simulink model "testBufferStorage3pt"  (R2018b)
settings: Solver=ode23  StartTime=0.0  StopTime=7000  MaxStep=300  RelTol=1e-3  EnableMultiTasking=on
undefined symbols (not defined in the file or in its folder): path_carnot
libraries: carnot x21, SignalEditorBlockLib x1
settings Model: Creator=drhf  LastModifiedBy=drhf
settings DataIOCC: LimitDataPoints=on  SaveFormat=Array
settings OptimizationCC: ExpressionDepthLimit=2147483647  LifeSpan=inf
settings DebuggingCC: UnderspecifiedInitializationDetection=Classic  MergeDetectMultiDrivingBlocksExec=none  SolverPrmCheckMsg=warning  StateNameClashWarn=warning  SFUnexpectedBacktrackingDiag=warning  SFNoUnconditionalDefaultTransitionDiag=warning  SFExecutionAtInitializationDiag=none
settings HardwareCC: ProdBitPerPointer=32  ProdBitPerSizeT=32  ProdBitPerPtrDiffT=32  ProdLargestAtomicFloat=None  ProdIntDivRoundTo=Undefined  ProdEndianess=Unspecified  ProdWordSize=32  ProdHWDeviceType=32-bit Generic
settings ModelReferenceCC: PropagateSignalLabelsOutOfModel=off
settings SFSimCC: SimUseLocalCustomCode=off
settings RTWCC: RTWUseLocalCustomCode=off
settings CodeAppCC: StateflowObjectComments=on
settings GRTTargetCC: TargetLangStandard=C89/C90 (ANSI)  GeneratePreprocessorConditionals=Disable all  CombineOutputUpdateFcns=off  GRTInterface=on
settings ConfigComp: CovMetricSettings=dw  CovHtmlReporting=on  CovSaveCumulativeToWorkspaceVar=on  CovSaveSingleToWorkspaceVar=on  CovExternalEMLEnable=off

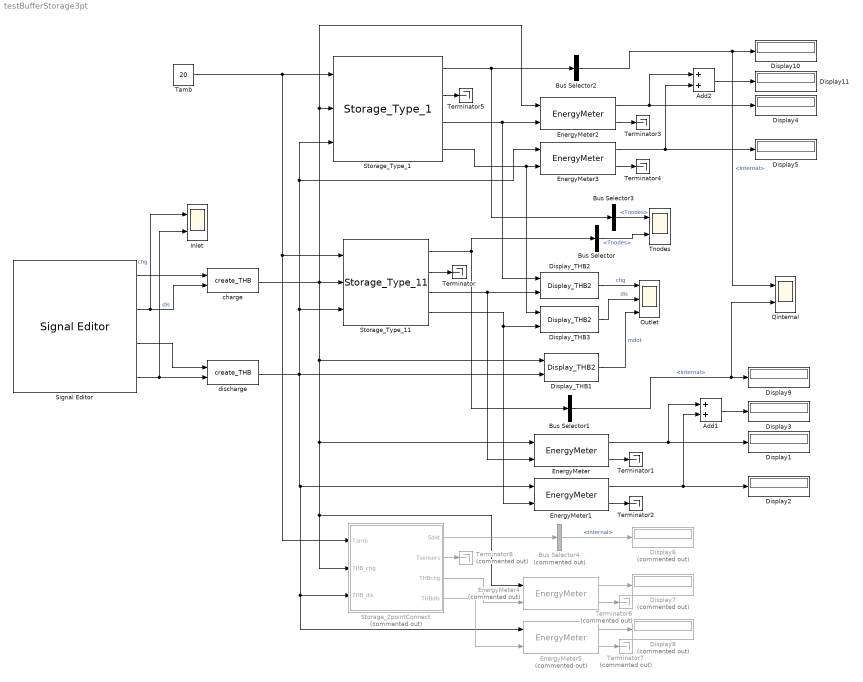
== system testBufferStorage3pt ==
  Add1 : Sum  Inputs=2
  Add2 : Sum  Inputs=2
  Bus Selector : BusSelector  OutputSignals=Tnodes
  Bus Selector1 : BusSelector  OutputSignals=energy.internal
  Bus Selector2 : BusSelector  OutputSignals=energy.internal
  Bus Selector3 : BusSelector  OutputSignals=Tnodes
  Bus Selector4 : BusSelector  Commented=on  OutputSignals=energy.internal
  Display{1..5,9..11} (8 alike) : Display
  Display6 : Display  Commented=on
  Display7 : Display  Commented=on
  Display8 : Display  Commented=on
  Display_THB1 : carnot/Outputs/Display_THB2  t=off  m=on  p=off  id=off  mix=off  d=off
      settings: SourceProductName=Carnot
  Display_THB2 : carnot/Outputs/Display_THB2  t=on  m=off  p=off  id=off  mix=off  d=off
      settings: SourceProductName=Carnot
  Display_THB3 : carnot/Outputs/Display_THB2  t=on  m=off  p=off  id=off  mix=off  d=off
      settings: SourceProductName=Carnot
  EnergyMeter{,1..3} (4 alike) : carnot/Control/EnergyMeter
      settings: SourceProductName=Carnot
  EnergyMeter4 : carnot/Control/EnergyMeter  Commented=on
      settings: SourceProductName=Carnot
  EnergyMeter5 : carnot/Control/EnergyMeter  Commented=on
      settings: SourceProductName=Carnot
  Inlet : Scope  NumInputPorts=2
  Outlet : Scope  NumInputPorts=3
  Qinternal : Scope  NumInputPorts=2
  Signal Editor : SignalEditorBlockLib/Signal Editor  FileName=storage3point_TestScenario.mat  ActiveScenario=Scenario  ActiveSignal=TDis  IsBus=off  OutputBusObjectStr=Bus: BusObject  SampleTime=0  ZeroCross=off  OutputAfterFinalValue=Setting to zero  Unit=inherit
  Storage_2pointConnect : Subsystem  Commented=on  mask(Buffer storage tank){t0=10, hgt=1.7684, stgtype=1, tini=[10 10 10 10 10 10 10 10 10 10], mpts=[1 2 3 4 5 6 7 8 9 10], PathName=fullfile(path_carnot('libsl'),'Storage','Thermal','Storage_Type_1','parameter_set'), FileName='StorageType1_500_L.mat', userPath=off, userParam=off, uwall=1, ubot=1, utop=1, axcond=1, volume=0.5, dia=0.6, standing=standing cylinder, nodes=10, mpoints=10, Tsensor=0.5, pipe1inlet=1, pipe1outlet=0, pipe1dia=0.03, pipe2inlet=0, pipe2outlet=1, pipe2dia=0.03}
      mask prompts: t0 "Initial temperature (vector or scalar) in °C"; hgt "Height of storage in m"; stgtype "Storage Type (0..5)"; tini "Start temperatures of nodes in °C"; mpts "Index to measured nodes"; PathName "Path"; FileName "Parameter set"; userPath "Edit path and name of parameter set"; userParam "User defined parameters"; uwall "Heat transfer coefficient to ambient [W/m²K]"; ubot "Heat transfer coefficient to ambient bottom [W/m²K]"; utop "Heat transfer coefficient to ambient top [W/m²K]"; axcond "Effective thermal conductivity [W/m/K]"; volume "Volume [m³]"; dia "Diameter [m]"; standing "Position"; nodes "Number of nodes"; mpoints "Number of node temperatures (for display)"; Tsensor "Temperature sensor position (0..1, 0 = bottom, 1 = top)"; pipe1inlet "relative height of inlet, range from 0 (= bottom) to 1 (= top)"; pipe1outlet "relative height of outlet, range from 0 (= bottom) to 1 (= top)"; pipe1dia "Diameter of pipe in m"; pipe2inlet "relative height of inlet, range from 0 (= bottom) to 1 (= top)"; pipe2outlet "relative height of outlet, range from 0 (= bottom) to 1 (= top)"; pipe2dia "Diameter of pipe in m"
      mask help:
      | Buffer storage for heating circuits. The storage model has the following components (with their typical position):
      | - one pipe connection for discharging (total height)
      | - one pipe connection for charging (total height)
      mask init:
      | [ok, param] = CarnotCallbacks_StorageConf('SetParam',stgtype,gcbh,PathName,FileName);
      mask Help: web(fullfile(path_carnot('help'),'Storage_Type_N.html'),'-helpbrowser')
      mask TypeOptions hgt: Pipe_Connection_1/hgt | Pipe_Connection_2/hgt
      mask TypeOptions stgtype: CreateSdat/stgtype
      mask TypeOptions tini: sfun_storageTnodes/tini
      mask TypeOptions mpts: select_T/Indices
      mask Callback userPath: [ok, param] = CarnotCallbacks_StorageConf('UserEdit',1,gcbh);
      mask Callback userParam: [ok, param] = CarnotCallbacks_StorageConf('UserEdit',1,gcbh);
      mask TypeOptions uwall: sfun_storageTnodes/uloss
      mask TypeOptions ubot: sfun_storageTnodes/ubot
      mask TypeOptions utop: sfun_storageTnodes/utop
      mask TypeOptions axcond: sfun_storageTnodes/cond
      mask TypeOptions volume: sfun_storageTnodes/volume | CreateSdat/volume
      mask TypeOptions dia: sfun_storageTnodes/dia | Pipe_Connection_1/dstg | Pipe_Connection_2/dstg
      mask TypeOptions standing: sfun_storageTnodes/standing
      mask TypeOptions nodes: sfun_storageTnodes/nodes | select_T/InputPortWidth | HX_EN12977_1/nodes | HX_EN12977_2/nodes | HX_EN12977_3/nodes | Pipe_Connection_1/nodes | Pipe_Connection_2/nodes | Pipe_Connection_3/nodes
      mask TypeOptions Tsensor: T_Sensor_Surface/pos
      mask TypeOptions pipe1inlet: Pipe_Connection_1/h_in
      mask TypeOptions pipe1outlet: Pipe_Connection_1/h_out
      mask TypeOptions pipe1dia: Pipe_Connection_1/dpipe
      mask TypeOptions pipe2inlet: Pipe_Connection_2/h_in
      mask TypeOptions pipe2outlet: Pipe_Connection_2/h_out
      mask TypeOptions pipe2dia: Pipe_Connection_2/dpipe
      mask DialogControl Container14 Prompt: Infos
      mask DialogControl ParameterGroupVar Prompt: Picking a parameter set
      mask DialogControl Control3 Prompt: Carnot public data
      mask DialogControl Control3 Callback: [ok, file] = CarnotCallbacks_StorageConf('GetFilename',1,gcbh,'public');
      mask DialogControl Control4 Prompt: Carnot internal data
      mask DialogControl Control4 Callback: [ok, file] = CarnotCallbacks_StorageConf('GetFilename',1,gcbh,'internal');
      mask DialogControl Control2 Prompt: Selected path
      mask DialogControl Control2 Callback: [ok, file] = CarnotCallbacks_StorageConf('GetFilename',1,gcbh,'selected');
      mask DialogControl Container4 Prompt: Parameter values
      mask DialogControl Container6 Prompt: Storage
      mask DialogControl Container8 Prompt: Connections
      mask DialogControl Container9 Prompt: Charging pipe
      mask DialogControl Container12 Prompt: Discharging pipe
      mask DialogControl Control6 Prompt: Save in Carnot internal data
      mask DialogControl Control6 Callback: [ok, param] = CarnotCallbacks_StorageConf('SaveFilename',1,gcbh,'internal','STG');
      mask DialogControl Control5 Prompt: Save in selected path
      mask DialogControl Control5 Callback: [ok, param] = CarnotCallbacks_StorageConf('SaveFilename',1,gcbh,'selected','STG');
      mask Display:
      | % user defined picture file
      | namestr = ['Storage_Type_', num2str(get_param(gcb,'stgtype'))];
      | picfile = fullfile(path_carnot('intlibsl'), 'Storage','Thermal', ...
      |     namestr,'parameter_set', [namestr, '.jpg']);
      | 
      | % show internal picture if defined
      | pic = false;
      | if  ~BlockIsInCarnotLibrary       % if not located in library
      |     if exist(picfile, 'file')
      |         image(imread(picfile), [0.25, 0, 0.45, 1])
      |         set_param(gcb, 'BackgroundColor', 'White')
      |         pic = true;
      |     end
      | end
      | 
      | % show public picture
      | if ~pic
      |     set_param(gcb, 'BackgroundColor', 'Red')
      | %     plot([40,30,30,40,60,70,70,60,40]/120+0.1,[90,80,10,0,0,10,80,90,90]/110+0.05, ...
      | %         [80,20]/120+0.1,[100,100]/110+0.05, ...
      | %         [50,50]/120+0.1,[90,100]/110+0.05, ...
      | %         [30,20]/120+0.1,[13,13]/110+0.05, ...
      | %         [80,70]/120+0.1,[13,13]/110+0.05)
      |       plot([40,30,30,40,60,70,70,60,40]/120+0.1,[90,80,20,10,10,20,80,90,90]/110+0.05, ...
      |            [80,20]/120+0.1,[100,100]/110+0.05, ...
      |            [50,50]/120+0.1,[90,100]/110+0.05, ...
      |            [80,20]/120+0.1,[0,0]/110+0.05, ...
      |            [50,50]/120+0.1,[0,10]/110+0.05)
      | end
  Storage_Type_1 : carnot/Storage/Thermal/Storage_Type_1  t0=10  hgt=1.7684  stgtype=1  tini=[10 10 10 10 10 10 10 10 10 10]  mpts=[1 2 3 4 5 6 7 8 9 10]  PathName=fullfile(path_carnot('libsl'),'Storage','Thermal','Storage_Type_1','parameter_set')  FileName='<user defined>'  userPath=off  userParam=on  uwall=1  ubot=1  utop=1  axcond=1  volume=0.5  dia=0.6  standing=standing cylinder  nodes=10  mpoints=10  Tsensor=0.5  pipe1inlet=1  pipe1outlet=0  pipe1dia=0.03  pipe2inlet=0.1  pipe2outlet=1  pipe2dia=0.03
      settings: SourceProductName=Carnot
  Storage_Type_11 : carnot/Storage/Thermal/Storage_Type_11  t0=10  hgt=1.7684  stgtype=11  tini=[10 10 10 10 10 10 10 10 10 10]  mpts=[1 2 3 4 5 6 7 8 9 10]  PathName='C:\Repos\carnot_svn\trunk\public\library_simulink\Storage\Thermal\Storage_Type_11\parameter_set\'  FileName='StorageType11_500_L.mat'  userPath=off  userParam=off  uwall=1  ubot=1  utop=1  axcond=1  volume=0.5  dia=0.6  standing=standing cylinder  nodes=10  mpoints=10  Tsensor=0.5  vTpiece=0.004  pipe1inlet=1  pipe1outlet=0  pipe1dia=0.03  pipe2inlet=0.1  pipe2outlet=1  pipe2dia=0.03
      settings: SourceProductName=Carnot
  Tamb : Constant  Value=20
  Terminator{,1..5} (6 alike) : Terminator
  Terminator6 : Terminator  Commented=on
  Terminator7 : Terminator  Commented=on
  Terminator8 : Terminator  Commented=on
  Tnodes : Scope  NumInputPorts=2
  charge : carnot/Source/Simple/create_THB  p=1e5  fluid=Water  mix=0  mix2=0  mix3=0  dia=0  hgt=0  mID=No Pressure Drop
      settings: SourceProductName=Carnot
  discharge : carnot/Source/Simple/create_THB  p=1e5  fluid=Water  mix=0  mix2=0  mix3=0  dia=0  hgt=0  mID=No Pressure Drop
      settings: SourceProductName=Carnot
  wires:
  Tamb/1 -> Storage_Type_1/1, Storage_Type_11/1, Storage_2pointConnect/1(Tamb)
  charge/1 -> Storage_Type_11/2, Storage_Type_1/2, EnergyMeter2/1, Storage_2pointConnect/2(THB_chg), EnergyMeter4/1, EnergyMeter/1, Display_THB1/1
  discharge/1 -> Storage_2pointConnect/3(THB_dis), EnergyMeter5/1, EnergyMeter1/1, Display_THB1/2, Storage_Type_11/3, Storage_Type_1/3, EnergyMeter3/1
  Storage_Type_11/3 -> EnergyMeter/2, Display_THB2/2
  Storage_Type_11/4 -> Display_THB3/2, EnergyMeter1/2
  Display_THB2/1 -> Outlet/1  "chg"
  Display_THB1/1 -> Outlet/3  "mdot"
  Storage_Type_11/2 -> Terminator/1
  Storage_Type_11/1 -> Bus Selector1/1, Bus Selector/1
  Bus Selector/1 -> Tnodes/2  "<Tnodes>"
  Bus Selector1/1 -> Qinternal/2, Display9/1  "<internal>"
  EnergyMeter/2 -> Terminator1/1
  EnergyMeter/1 -> Add1/1, Display1/1
  EnergyMeter1/1 -> Add1/2, Display2/1
  EnergyMeter1/2 -> Terminator2/1
  Storage_Type_1/1 -> Bus Selector3/1, Bus Selector2/1
  Storage_Type_1/2 -> Terminator5/1
  Storage_Type_1/3 -> Display_THB2/1, EnergyMeter2/2
  Storage_Type_1/4 -> Display_THB3/1, EnergyMeter3/2
  Bus Selector3/1 -> Tnodes/1  "<Tnodes>"
  EnergyMeter5/2 -> Terminator7/1
  EnergyMeter5/1 -> Display8/1
  EnergyMeter4/1 -> Display7/1
  EnergyMeter4/2 -> Terminator6/1
  Bus Selector4/1 -> Display6/1  "<internal>"
  Storage_2pointConnect/1(Sdat) -> Bus Selector4/1
  Storage_2pointConnect/2(Tsensors) -> Terminator8/1
  Storage_2pointConnect/3(THBchg) -> EnergyMeter4/2
  Storage_2pointConnect/4(THBdis) -> EnergyMeter5/2
  Bus Selector2/1 -> Qinternal/1, Display10/1  "<internal>"
  EnergyMeter3/1 -> Add2/2, Display5/1
  EnergyMeter3/2 -> Terminator4/1
  EnergyMeter2/1 -> Add2/1, Display4/1
  EnergyMeter2/2 -> Terminator3/1
  Add1/1 -> Display3/1
  Add2/1 -> Display11/1
  Signal Editor/1 -> charge/1
  Signal Editor/3 -> discharge/1
  Signal Editor/2 -> Inlet/1, charge/2  "chg"
  Signal Editor/4 -> Inlet/2, discharge/2  "dis"
  Display_THB3/1 -> Outlet/2  "dis"

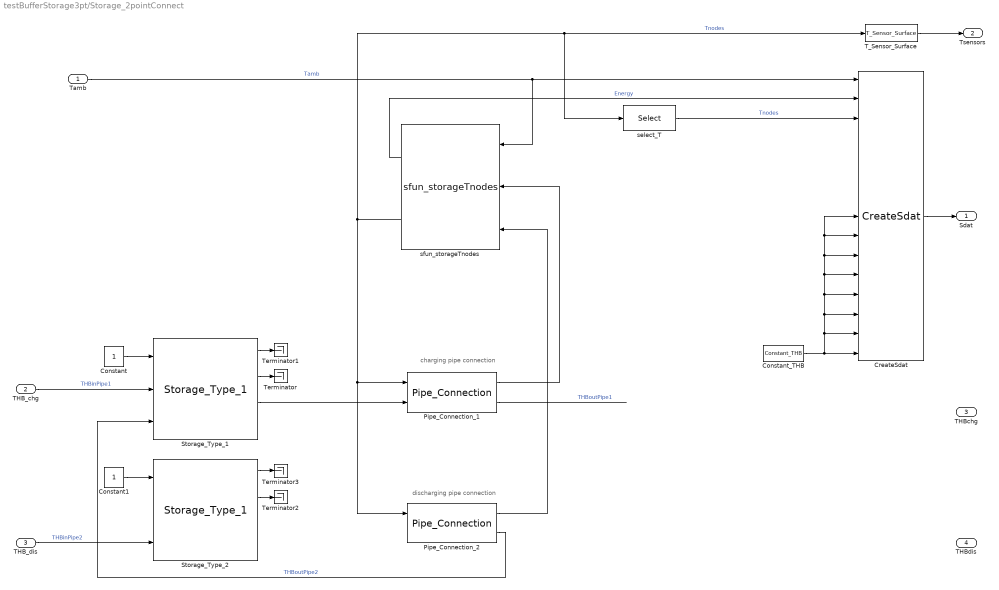
== system testBufferStorage3pt/Storage_2pointConnect ==
  note: discharging pipe connection
  note: charging pipe connection
  Tamb : Inport
  THB_chg : Inport  Port=2
  THB_dis : Inport  Port=3
  Constant : Constant
  Constant1 : Constant
  Constant_THB : carnot/Source/Simple/Constant_THB  t=20  mdot=0  p=1e5  mID=No Pressure Drop  fluid=Water  mix=0  mix2=0  mix3=0  dia=0.02  hgt=0
      settings: SourceProductName=Carnot
  CreateSdat : carnot/Basic/Thermal_Models/CreateSdat  volume=volume  stgtype=stgtype
      settings: SourceProductName=Carnot
  Pipe_Connection_1 : carnot/Storage/Thermal/Storage_Ports/Pipe_Connection  h_in=pipe1inlet  h_out=pipe1outlet  hgt=hgt  dpipe=pipe1dia  dstg=dia  height=-1.7684  nodes=nodes
      settings: SourceProductName=Carnot
  Pipe_Connection_2 : carnot/Storage/Thermal/Storage_Ports/Pipe_Connection  h_in=pipe2inlet  h_out=pipe2outlet  hgt=hgt  dpipe=pipe2dia  dstg=dia  height=1.7684  nodes=nodes
      settings: SourceProductName=Carnot
  Storage_Type_1 : carnot/Storage/Thermal/Storage_Type_1  t0=10  hgt=0.63662  stgtype=1  tini=10  mpts=1  PathName=fullfile(path_carnot('libsl'),'Storage','Thermal','Storage_Type_1','parameter_set')  FileName='<user defined>'  userPath=off  userParam=on  uwall=0  ubot=0  utop=0  axcond=0  volume=0.005  dia=0.1  standing=standing cylinder  nodes=1  mpoints=1  Tsensor=0.5  pipe1inlet=1  pipe1outlet=0  pipe1dia=0.03  pipe2inlet=0  pipe2outlet=1  pipe2dia=0.03
      settings: SourceProductName=Carnot
  Storage_Type_2 : carnot/Storage/Thermal/Storage_Type_1  t0=10  hgt=0.63662  stgtype=1  tini=10  mpts=1  PathName=fullfile(path_carnot('libsl'),'Storage','Thermal','Storage_Type_1','parameter_set')  FileName='<user defined>'  userPath=off  userParam=on  uwall=0  ubot=0  utop=0  axcond=0  volume=0.005  dia=0.1  standing=standing cylinder  nodes=1  mpoints=1  Tsensor=0.5  pipe1inlet=1  pipe1outlet=0  pipe1dia=0.03  pipe2inlet=0  pipe2outlet=1  pipe2dia=0.03
      settings: SourceProductName=Carnot
  T_Sensor_Surface : carnot/Control/T_Sensor_Surface  pos=Tsensor  tdel=10  t0=mean(tini)
      settings: SourceProductName=Carnot
  Terminator{,1..3} (4 alike) : Terminator
  select_T : Selector  InputPortWidth=nodes  IndexOptions=Index vector (dialog)  Indices=[1 2 3 4 5 6 7 8 9 10]  OutputSizes=1
  sfun_storageTnodes : carnot/Basic/Thermal_Models/sfun_storageTnodes  uloss=uwall  ubot=ubot  utop=utop  cond=axcond  volume=volume  dia=dia  standing=standing cylinder  tini=tini  nodes=nodes  nconnect=2  elimthermocline=2  condinvtc=1e5
      settings: SourceProductName=Carnot
  Sdat : Outport
  Tsensors : Outport  Port=2
  THBchg : Outport  Port=3
  THBdis : Outport  Port=4
  wires:
  Constant_THB/1 -> CreateSdat/15, CreateSdat/8, CreateSdat/9, CreateSdat/10, CreateSdat/11, CreateSdat/12, CreateSdat/13, CreateSdat/14
  T_Sensor_Surface/1 -> Tsensors/1
  Pipe_Connection_1/1 -> sfun_storageTnodes/2
  ? -> THBchg/1, CreateSdat/5  "THBoutPipe1"
  CreateSdat/1 -> Sdat/1
  sfun_storageTnodes/2 -> Pipe_Connection_2/1, Pipe_Connection_1/1, T_Sensor_Surface/1, select_T/1  "Tnodes"
  select_T/1 -> CreateSdat/3  "Tnodes"
  Tamb/1 -> CreateSdat/1, sfun_storageTnodes/1  "Tamb"
  THB_dis/1 -> Storage_Type_2/3  "THBinPipe2"
  Pipe_Connection_2/1 -> sfun_storageTnodes/3
  sfun_storageTnodes/1 -> CreateSdat/2  "Energy"
  THB_chg/1 -> Storage_Type_1/2  "THBinPipe1"
  ? -> THBdis/1, CreateSdat/7  "THBoutPipe2"
  Pipe_Connection_1/2 -> ?  "THBoutPipe1"
  Pipe_Connection_2/2 -> Storage_Type_1/3  "THBoutPipe2"
  Constant/1 -> Storage_Type_1/1
  Storage_Type_1/2 -> Terminator/1
  Storage_Type_1/1 -> Terminator1/1
  Constant1/1 -> Storage_Type_2/1
  Storage_Type_2/2 -> Terminator2/1
  Storage_Type_2/1 -> Terminator3/1
  Storage_Type_1/3 -> Pipe_Connection_1/2
